simulink model "ex2_2"  (R2025b)
settings: Solver=VariableStepAuto  StartTime=0.0  StopTime=700  RelTol=1e-3
libraries: simulink x1
settings Model: Creator=rares  LastModifiedBy=rares

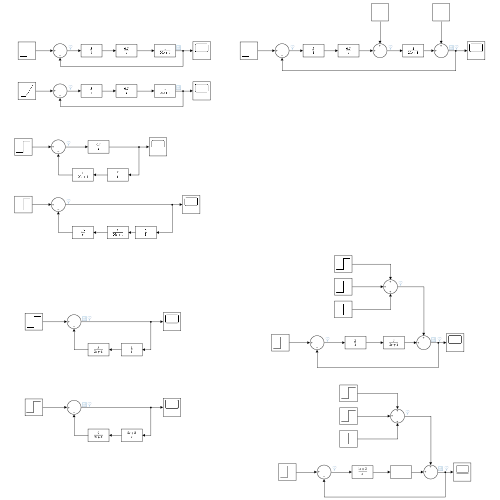
[thumbnail: Simulink's stored preview of the top-level diagram]
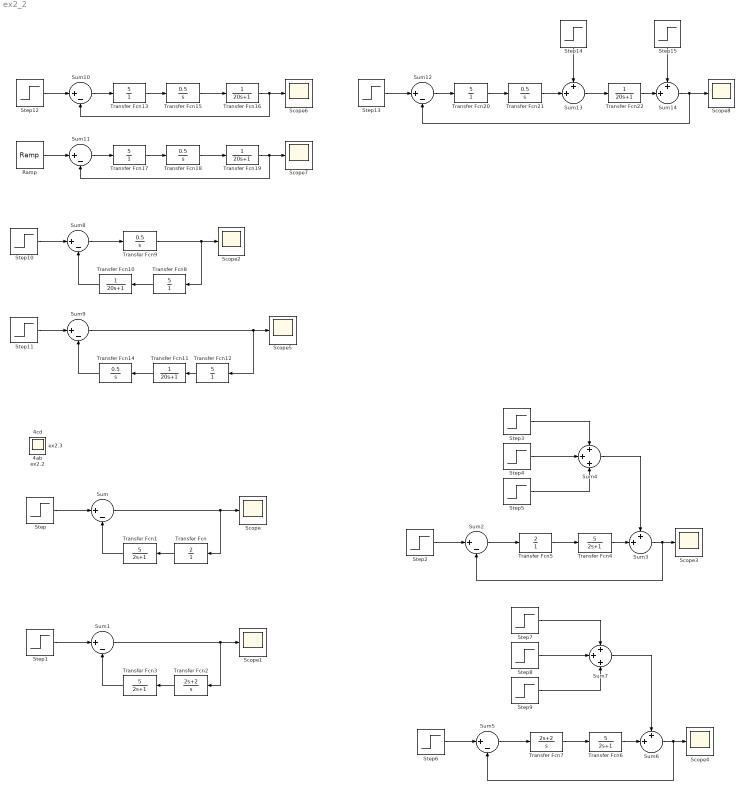
== system ex2_2 ==
  Ramp : simulink/Sources/Ramp  slope=1  start=0  InitialOutput=0
  Scope{,1..8} (9 alike) : Scope
      Scope settings: ActiveDisplayYMinimum=-1  ActiveDisplayYMaximum=1
      Scope1 settings: ActiveDisplayYMinimum=-1  ActiveDisplayYMaximum=1
      Scope2 settings: ActiveDisplayYMinimum=-1  ActiveDisplayYMaximum=1  DataLoggingVariableName=ScopeData6
      Scope3 settings: ActiveDisplayYMinimum=-1  ActiveDisplayYMaximum=1  DataLoggingVariableName=ScopeData3
      Scope4 settings: ActiveDisplayYMinimum=-1  ActiveDisplayYMaximum=1  DataLoggingVariableName=ScopeData4
      Scope5 settings: ActiveDisplayYMinimum=-1  ActiveDisplayYMaximum=1  DataLoggingVariableName=ScopeData7
      Scope6 settings: ActiveDisplayYMinimum=-1  ActiveDisplayYMaximum=1  DataLoggingVariableName=ScopeData9
      Scope7 settings: ActiveDisplayYMinimum=-1  ActiveDisplayYMaximum=1  DataLoggingVariableName=ScopeData10
      Scope8 settings: ActiveDisplayYMinimum=-1  ActiveDisplayYMaximum=1  DataLoggingVariableName=ScopeData11
  Step{,1..2,6,12..13} (6 alike) : Step  SampleTime=0
  Step10 : Step  Time=150  After=0.2  SampleTime=0
  Step11 : Step  Time=450  After=0.1  SampleTime=0
  Step14 : Step  Time=150  After=0.2  SampleTime=0
  Step15 : Step  Time=450  After=0.1  SampleTime=0
  Step3 : Step  Time=30  After=0.2  SampleTime=0
  Step4 : Step  Time=60  After=0.3  SampleTime=0
  Step5 : Step  Time=90  After=0.4  SampleTime=0
  Step7 : Step  Time=30  After=0.2  SampleTime=0
  Step8 : Step  Time=60  After=0.3  SampleTime=0
  Step9 : Step  Time=90  After=0.4  SampleTime=0
  Sum{,1..2,5,8..12} (9 alike) : Sum  Inputs=|+-
  Sum{3,6,13..14} (4 alike) : Sum  Inputs=++|
  Sum4 : Sum  Inputs=+++
  Sum7 : Sum  Inputs=+++
  Transfer Fcn : TransferFcn  Numerator=[2]  Denominator=[1]
  Transfer Fcn{1,3..4,6} (4 alike) : TransferFcn  Numerator=[5]  Denominator=[2 1]
  Transfer Fcn{10..11,16,19,22} (5 alike) : TransferFcn  Denominator=[20 1]
  Transfer Fcn{8,12..13,17,20} (5 alike) : TransferFcn  Numerator=[5]  Denominator=[1]
  Transfer Fcn{9,14..15,18,21} (5 alike) : TransferFcn  Numerator=[0.5]  Denominator=[1 0]
  Transfer Fcn2 : TransferFcn  Numerator=[2 2]  Denominator=[1 0]
  Transfer Fcn5 : TransferFcn  Numerator=[2]  Denominator=[1]
  Transfer Fcn7 : TransferFcn  Numerator=[2 2]  Denominator=[1 0]
  4ab : Scope
      settings: ActiveDisplayYMinimum=-1  ActiveDisplayYMaximum=1  DataLoggingVariableName=ScopeData8
  4cd : Scope
      settings: ActiveDisplayYMinimum=-0.224915507642718  ActiveDisplayYMaximum=2.0242395687844628  DataLoggingVariableName=ScopeData12
  ex2.2 : Scope
      settings: ActiveDisplayYMinimum=-0.1798479755633775  ActiveDisplayYMaximum=1.1310942195070419  DataLoggingVariableName=ScopeData2
  ex2.3 : Scope
      settings: ActiveDisplayYMinimum=-1  ActiveDisplayYMaximum=1  DataLoggingVariableName=ScopeData5
  wires:
  Step/1 -> Sum/1
  Sum/1 -> Transfer Fcn/1, Scope/1
  Transfer Fcn/1 -> Transfer Fcn1/1
  Transfer Fcn1/1 -> Sum/2
  Transfer Fcn2/1 -> Transfer Fcn3/1
  Transfer Fcn3/1 -> Sum1/2
  Step1/1 -> Sum1/1
  Sum1/1 -> Transfer Fcn2/1, Scope1/1
  Step2/1 -> Sum2/1
  Sum2/1 -> Transfer Fcn5/1
  Transfer Fcn5/1 -> Transfer Fcn4/1
  Transfer Fcn4/1 -> Sum3/2
  Sum3/1 -> Sum2/2, Scope3/1
  Step3/1 -> Sum4/1
  Step4/1 -> Sum4/2
  Step5/1 -> Sum4/3
  Sum4/1 -> Sum3/1
  Step7/1 -> Sum7/1
  Step9/1 -> Sum7/3
  Sum7/1 -> Sum6/1
  Sum5/1 -> Transfer Fcn7/1
  Step8/1 -> Sum7/2
  Step6/1 -> Sum5/1
  Transfer Fcn7/1 -> Transfer Fcn6/1
  Transfer Fcn6/1 -> Sum6/2
  Sum6/1 -> Sum5/2, Scope4/1
  Step10/1 -> Sum8/1
  Sum8/1 -> Transfer Fcn9/1
  Transfer Fcn9/1 -> Transfer Fcn8/1, Scope2/1
  Transfer Fcn8/1 -> Transfer Fcn10/1
  Transfer Fcn10/1 -> Sum8/2
  Step11/1 -> Sum9/1
  Transfer Fcn12/1 -> Transfer Fcn11/1
  Sum9/1 -> Transfer Fcn12/1, Scope5/1
  Transfer Fcn11/1 -> Transfer Fcn14/1
  Transfer Fcn14/1 -> Sum9/2
  Step12/1 -> Sum10/1
  Sum10/1 -> Transfer Fcn13/1
  Transfer Fcn13/1 -> Transfer Fcn15/1
  Transfer Fcn15/1 -> Transfer Fcn16/1
  Transfer Fcn16/1 -> Sum10/2, Scope6/1
  Transfer Fcn19/1 -> Scope7/1, Sum11/2
  Transfer Fcn18/1 -> Transfer Fcn19/1
  Transfer Fcn17/1 -> Transfer Fcn18/1
  Sum11/1 -> Transfer Fcn17/1
  Ramp/1 -> Sum11/1
  Transfer Fcn20/1 -> Transfer Fcn21/1
  Sum12/1 -> Transfer Fcn20/1
  Step13/1 -> Sum12/1
  Sum13/1 -> Transfer Fcn22/1
  Transfer Fcn21/1 -> Sum13/2
  Transfer Fcn22/1 -> Sum14/2
  Sum14/1 -> Sum12/2, Scope8/1
  Step14/1 -> Sum13/1
  Step15/1 -> Sum14/1
